simulink model "sim_linear_control_old"  (R2018a)
settings: Solver=ode3  StartTime=0.0  StopTime=1  FixedStep=0.001  RelTol=1e-3
values from neighbouring files (symbols this model uses):
  C = [1 0 ... (first row only)    [lin_control.m]    (also in lin_control3.m = [0 1])
  CA = C*A    [lin_control.m]    (also in lin_control3.m)
  invCB = pinv(C*B)    [lin_control.m]    (also in lin_control3.m)
settings Model: Creator=E183308  LastModifiedBy=E183308

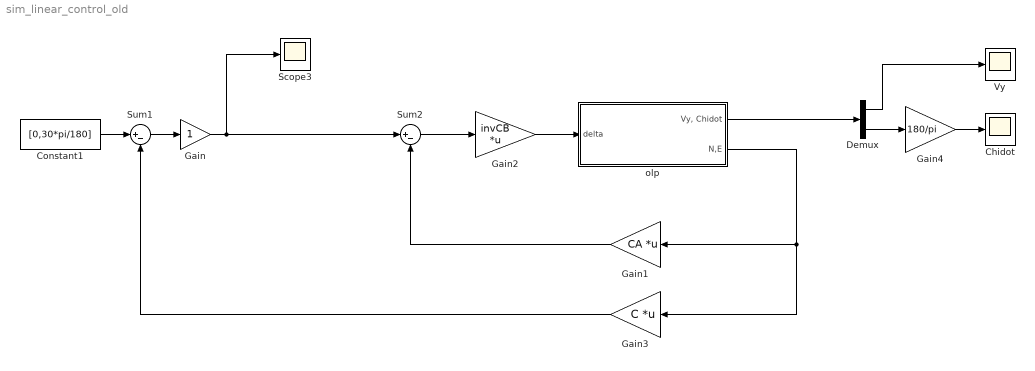
== system sim_linear_control_old ==
  Chidot : Scope
  Constant1 : Constant  Value=[0,30*pi/180]
  Demux : Demux  Outputs=2
  Gain : Gain
  Gain1 : Gain  Gain=CA  Multiplication=Matrix(K*u)
  Gain2 : Gain  Gain=invCB  Multiplication=Matrix(K*u)
  Gain3 : Gain  Gain=C  Multiplication=Matrix(K*u)
  Gain4 : Gain  Gain=180/pi
  Scope3 : Scope
  Sum1 : Sum  Inputs=|+-
  Sum2 : Sum  Inputs=|+-
  Vy : Scope
  olp : Subsystem
  wires:
  Sum1/1 -> Gain/1
  Constant1/1 -> Sum1/1
  Sum2/1 -> Gain2/1
  Gain1/1 -> Sum2/2
  Gain/1 -> Scope3/1, Sum2/1
  Gain2/1 -> olp/1(delta)
  olp/2(N,E) -> Gain3/1, Gain1/1
  Gain3/1 -> Sum1/2
  olp/1("Vy, Chidot") -> Demux/1
  Demux/1 -> Vy/1
  Demux/2 -> Gain4/1
  Gain4/1 -> Chidot/1

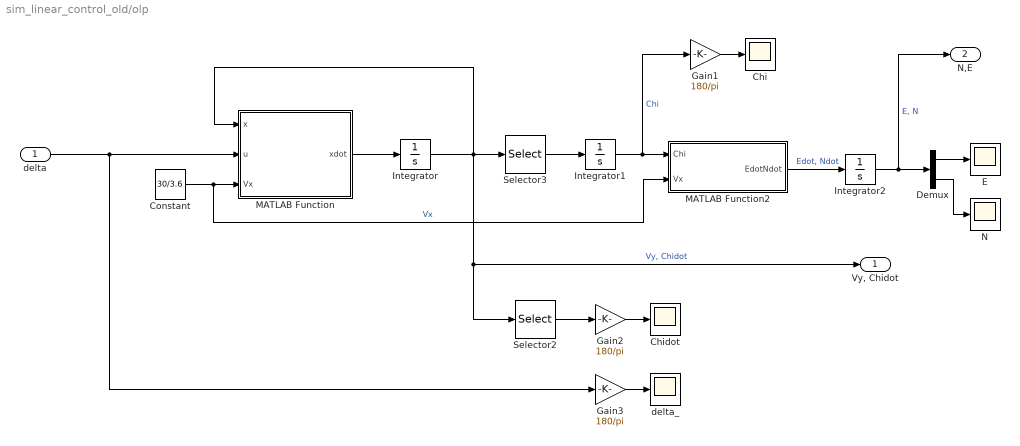
== system sim_linear_control_old/olp ==
  delta : Inport
  Chi : Scope
  Chidot : Scope
  Constant : Constant  Value=30/3.6
  Demux : Demux  Outputs=2
  E : Scope
  Gain1 : Gain  Gain=180/pi
  Gain2 : Gain  Gain=180/pi
  Gain3 : Gain  Gain=180/pi
  Integrator : Integrator  InitialCondition=[0;0]
  Integrator1 : Integrator
  Integrator2 : Integrator  InitialCondition=[0;0]
  MATLAB Function : MATLAB Function  TreatAsAtomicUnit=on
  MATLAB Function2 : MATLAB Function  TreatAsAtomicUnit=on
  N : Scope
  Selector2 : Selector  InputPortWidth=2  IndexOptions=Index vector (dialog)  Indices=2  OutputSizes=1
  Selector3 : Selector  InputPortWidth=2  IndexOptions=Index vector (dialog)  Indices=2  OutputSizes=1
  delta_ : Scope
  "Vy, Chidot" : Outport
  N,E : Outport  Port=2
  wires:
  Gain2/1 -> Chidot/1
  Integrator1/1 -> Gain1/1, MATLAB Function2/1(Chi)  "Chi"
  Selector2/1 -> Gain2/1
  Selector3/1 -> Integrator1/1
  Integrator/1 -> Selector2/1, "Vy, Chidot"/1, MATLAB Function/1(x), Selector3/1  "Vy, Chidot"
  Gain3/1 -> delta_/1
  MATLAB Function2/1(EdotNdot) -> Integrator2/1  "Edot, Ndot"
  Integrator2/1 -> N,E/1, Demux/1  "E, N"
  Gain1/1 -> Chi/1
  Demux/2 -> N/1
  delta/1 -> Gain3/1, MATLAB Function/2(u)
  Constant/1 -> MATLAB Function2/2(Vx), MATLAB Function/3(Vx)  "Vx"
  Demux/1 -> E/1
  MATLAB Function/1(xdot) -> Integrator/1

== matlab function sim_linear_control_old/olp/MATLAB Function ==
  data: x input; u input; xdot output; Vx input
function xdot = dynamic_lin(x,u,Vx)

% sports sedan

m = 1724; % kg
Iz = 3400; % kg/m^2
a = 1.35; % m
b = 1.15; % m
Cf = 12*1e4; % N/rad
Cr = 175*1e3; % N/rad
mu = 0.5225;

% x = [vy Chidot], u = delta

A = [-(Cf+Cr)/m  -(a*Cf-b*Cr)/(m*Vx)-Vx; 
    -(a*Cf-b*Cr)/Iz -(a^2*Cf-b^2*Cr)/(Iz*Vx)];

B = [Cf/m; a*Cf/Iz];

xdot = A*x + B*u;

== matlab function sim_linear_control_old/olp/MATLAB Function2 ==
  data: Chi input; EdotNdot output; Vx input
function EdotNdot = kinematics(Chi,Vx)

Edot = Vx*sin(Chi);
Ndot = Vx*cos(Chi);

EdotNdot = [Edot; Ndot];
